simulink model "Modele_NLin_BO"  (R2018a)
settings: Solver=ode45  StartTime=0.0  StopTime=100  RelTol=1e-3  EnableMultiTasking=on
values from neighbouring files (symbols this model uses):
  Jt = 5.8743e-04    (= 0.00058743)    [parametres.m]
  k = 0.0337    [parametres.m]
  Kp = 10/6.28    (= 1.5923566879)    [parametres.m]
  Kv = 0.0497    [parametres.m]
  Pente = 8.7060e-10    (= 8.706e-10)    [parametres.m]
  R = 5.8    [parametres.m]
  ro = 1/20    (= 0.05)    [parametres.m]
libraries: simulink x1
settings Model: Creator=reamaa  LastModifiedBy=Georges Salloum
settings DataIOCC: LimitDataPoints=on  SaveFormat=Array  SignalLoggingSaveFormat=ModelDataLogs
settings OptimizationCC: BlockReduction=off  BooleanDataType=off  InitFltsAndDblsToZero=on  LifeSpan=inf
settings DebuggingCC: SaveWithParameterizedLinksMsg=none  UnderspecifiedInitializationDetection=Classic  MergeDetectMultiDrivingBlocksExec=none  SignalResolutionControl=TryResolveAllWithWarning  MultiTaskDSMMsg=warning  MultiTaskCondExecSysMsg=none  FcnCallInpInsideContextMsg=warning  SFUnexpectedBacktrackingDiag=warning  SFNoUnconditionalDefaultTransitionDiag=warning  SFExecutionAtInitializationDiag=none
settings HardwareCC: ProdBitPerPointer=32  ProdBitPerSizeT=32  ProdBitPerPtrDiffT=32  ProdLargestAtomicFloat=None  ProdIntDivRoundTo=Undefined  ProdEndianess=Unspecified  ProdWordSize=32  ProdHWDeviceType=32-bit Generic  TargetUnknown=on
settings ModelReferenceCC: PropagateSignalLabelsOutOfModel=off
settings CodeAppCC: StateflowObjectComments=on
settings GRTTargetCC: TargetFcnLib=ansi_tfl_tmw.mat  TargetLangStandard=C89/C90 (ANSI)  CombineOutputUpdateFcns=off  GRTInterface=on
settings ConfigComp: CovMetricSettings=dw  CovSaveCumulativeToWorkspaceVar=on  CovSaveSingleToWorkspaceVar=on  CovExternalEMLEnable=off

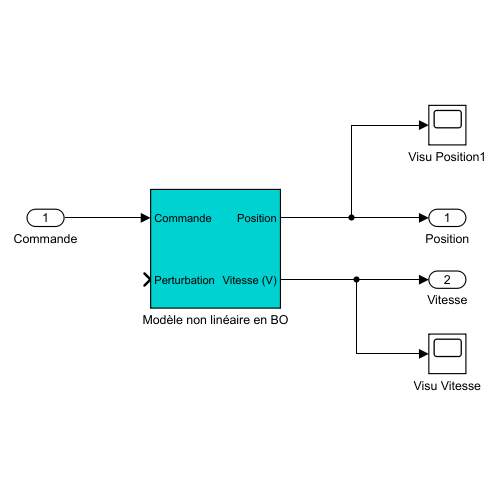
[thumbnail: Simulink's stored preview of the top-level diagram]
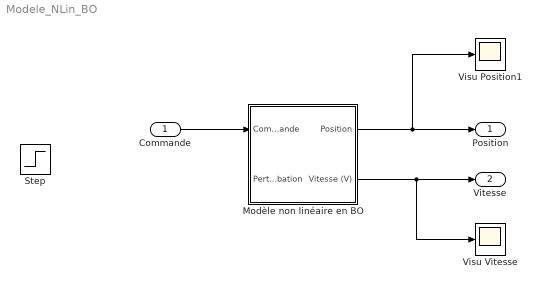
== system Modele_NLin_BO ==
  Commande : Inport
  Modèle non linéaire en BO : Subsystem
  Visu Position1 : Scope
  Visu Vitesse : Scope
  Position : Outport
  Vitesse : Outport  Port=2
  Step : Step  IOType=siggen  SampleTime=0
  wires:
  Modèle non linéaire en BO/1(Position) -> Visu Position1/1, Position/1
  Modèle non linéaire en BO/2(Vitesse (V)) -> Visu Vitesse/1, Vitesse/1
  Commande/1 -> Modèle non linéaire en BO/1(Commande)

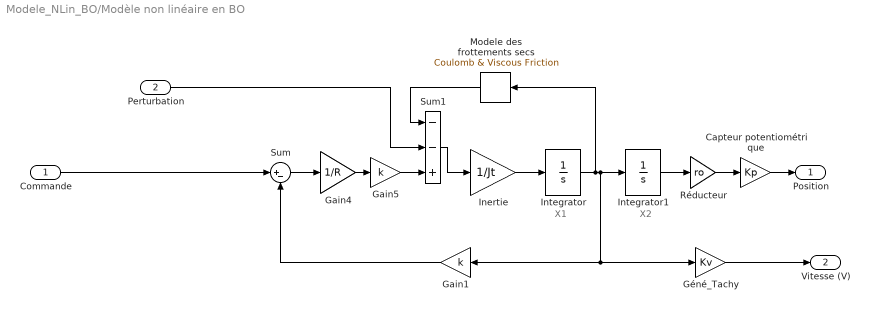
== system Modele_NLin_BO/Modèle non linéaire en BO ==
  note: X1
  note: X2
  Commande : Inport
  Perturbation : Inport  Port=2
  Capteur potentiométrique : Gain  Gain=Kp  SaturateOnIntegerOverflow=on  OutDataTypeStr=Inherit: Same as input  ParamDataTypeStr=Inherit: Same as input
  Gain1 : Gain  Gain=k  SaturateOnIntegerOverflow=on  OutDataTypeStr=Inherit: Same as input  ParamDataTypeStr=Inherit: Same as input
  Gain4 : Gain  Gain=1/R  SaturateOnIntegerOverflow=on  OutDataTypeStr=Inherit: Same as input  ParamDataTypeStr=Inherit: Same as input
  Gain5 : Gain  Gain=k  SaturateOnIntegerOverflow=on  OutDataTypeStr=Inherit: Same as input  ParamDataTypeStr=Inherit: Same as input
  Géné_Tachy : Gain  Gain=Kv  SaturateOnIntegerOverflow=on  OutDataTypeStr=Inherit: Same as input  ParamDataTypeStr=Inherit: Same as input
  Inertie : Gain  Gain=1/Jt  SaturateOnIntegerOverflow=on  OutDataTypeStr=Inherit: Same as input  ParamDataTypeStr=Inherit: Same as input
  Integrator : Integrator
  Integrator1 : Integrator
  Modele des frottements secs : simulink/Discontinuities/Coulomb & Viscous Friction  offset=Csec  gain=Pente
  Réducteur : Gain  Gain=ro  OutDataTypeStr=Inherit: Same as input  ParamDataTypeStr=Inherit: Same as input
  Sum : Sum  Inputs=|+-  InputSameDT=on  SaturateOnIntegerOverflow=on  OutDataTypeStr=Inherit: Same as first input
  Sum1 : Sum  Inputs=--+  InputSameDT=on  SaturateOnIntegerOverflow=on  OutDataTypeStr=Inherit: Same as first input
  Position : Outport
  Vitesse (V) : Outport  Port=2
  wires:
  Géné_Tachy/1 -> Vitesse (V)/1
  Capteur potentiométrique/1 -> Position/1
  Sum1/1 -> Inertie/1
  Réducteur/1 -> Capteur potentiométrique/1
  Integrator1/1 -> Réducteur/1
  Gain1/1 -> Sum/2
  Integrator/1 -> Géné_Tachy/1, Gain1/1, Integrator1/1, Modele des frottements secs/1
  Inertie/1 -> Integrator/1
  Gain4/1 -> Gain5/1
  Sum/1 -> Gain4/1
  Gain5/1 -> Sum1/3
  Perturbation/1 -> Sum1/2
  Commande/1 -> Sum/1
  Modele des frottements secs/1 -> Sum1/1
